simulink model "NonLinear_MotorControl"  (R2017b)
settings: Solver=ode4  StartTime=0.0  StopTime=10  FixedStep=0.0001  MaxStep=0.001  MinStep=0.0001  RelTol=1e-3
(part 2 of 2)

== matlab function NonLinear_MotorControl/System Dynamics/MATLAB Function ==
  data: q input; tau input; q_ddot output; q_dot input
function q_ddot = fcn(q,tau,q_dot)
   q_1 = q(1);
   q_2 = q(2);
   q_3 = q(3);
   q_4 = q(4);
   q_5 = q(5);
   %% M
   M = ...
[                                                                                                                                                                                                                                                                                                                                                                                                                                                                                                                                                                                                                                                                                                                                                                                                               243/2,                                                                                                                                                                                                                               (1637253847765431*cos(q_2 + q_4 + q_5))/2748779069440 + (3015813*sin(q_2 + q_4 + q_5))/12500 + (1637253847765431*cos(q_2 + q_4 - q_5))/2748779069440 + (3015813*sin(q_2 + q_4 - q_5))/12500 - (1637253847765431*cos(q_2 + q_4))/1374389534720 + (13930449*cos(q_2))/500000 + (11396226878722115871*sin(q_2))/1759218604441600 - (1637253847765431*2^(1/2)*cos(q_2 + q_4 - q_5))/2748779069440 - (3015813*2^(1/2)*sin(q_2 + q_4 - q_5))/25000 - (3567380807909369503983*2^(1/2)*cos(q_2 + q_4))/2199023255552000000 + (1637253847765431*2^(1/2)*cos(q_2 + q_4 + q_5))/2748779069440 + (3015813*2^(1/2)*sin(q_2 + q_4 + q_5))/25000,                                                                            0,                                                                                                                                                                                                                                                                                                               (1637253847765431*cos(q_2 + q_4 + q_5))/2748779069440 + (3015813*sin(q_2 + q_4 + q_5))/12500 + (1637253847765431*cos(q_2 + q_4 - q_5))/2748779069440 + (3015813*sin(q_2 + q_4 - q_5))/12500 - (1637253847765431*cos(q_2 + q_4))/1374389534720 - (1637253847765431*2^(1/2)*cos(q_2 + q_4 - q_5))/2748779069440 - (3015813*2^(1/2)*sin(q_2 + q_4 - q_5))/25000 - (3567380807909369503983*2^(1/2)*cos(q_2 + q_4))/2199023255552000000 + (1637253847765431*2^(1/2)*cos(q_2 + q_4 + q_5))/2748779069440 + (3015813*2^(1/2)*sin(q_2 + q_4 + q_5))/25000,                                                                                           (1637253847765431*cos(q_2 + q_4 + q_5))/2748779069440 + (3015813*sin(q_2 + q_4 + q_5))/12500 - (1637253847765431*cos(q_2 + q_4 - q_5))/2748779069440 - (3015813*sin(q_2 + q_4 - q_5))/12500 + (1637253847765431*2^(1/2)*cos(q_2 + q_4 - q_5))/2748779069440 + (3015813*2^(1/2)*sin(q_2 + q_4 - q_5))/25000 + (1637253847765431*2^(1/2)*cos(q_2 + q_4 + q_5))/2748779069440 + (3015813*2^(1/2)*sin(q_2 + q_4 + q_5))/25000
  (13930449*cos(q_2))/500000 + (11396226878722115871*sin(q_2))/1759218604441600 - (1637253847765431*cos(q_2)*cos(q_4))/1374389534720 + (1637253847765431*sin(q_2)*sin(q_4))/1374389534720 - (3567380807909369503983*2^(1/2)*cos(q_2)*cos(q_4))/2199023255552000000 + (3567380807909369503983*2^(1/2)*sin(q_2)*sin(q_4))/2199023255552000000 + (1637253847765431*cos(q_2)*cos(q_4)*cos(q_5))/1374389534720 + (3015813*cos(q_2)*cos(q_5)*sin(q_4))/6250 + (3015813*cos(q_4)*cos(q_5)*sin(q_2))/6250 - (1637253847765431*cos(q_5)*sin(q_2)*sin(q_4))/1374389534720 + (3015813*2^(1/2)*cos(q_2)*cos(q_4)*sin(q_5))/12500 - (1637253847765431*2^(1/2)*cos(q_2)*sin(q_4)*sin(q_5))/1374389534720 - (1637253847765431*2^(1/2)*cos(q_4)*sin(q_2)*sin(q_5))/1374389534720 - (3015813*2^(1/2)*sin(q_2)*sin(q_4)*sin(q_5))/12500,  sin(q_5)/1000 - (47028073017942265058105238873*cos(q_5))/151115727451828646838272 - (1637253847765431*sin(q_4))/1374389534720 - (57*sin(2*q_5))/2000 - (86625503688717695659*2^(1/2)*sin(2*q_5))/2748779069440000 - (3015813*cos(q_4)*cos(q_5))/6250 + (1637253847765431*cos(q_5)*sin(q_4))/1374389534720 - (25261205975153249495668933896699961*cos(q_5)^2)/118059162071741130342400000000 + (21357421969732009*2^(1/2))/549755813888 + (3796988859053507*2^(1/2)*cos(q_5))/549755813888 - (3567380807909369503983*2^(1/2)*sin(q_4))/2199023255552000000 - (86625502314328160939*2^(1/2)*sin(q_5))/1374389534720000 - (16938612281049*2^(1/2)*cos(q_5)^2)/68719476736 + (1637253847765431*2^(1/2)*cos(q_4)*sin(q_5))/1374389534720 + (3015813*2^(1/2)*sin(q_4)*sin(q_5))/12500 + 31233135728824415250615508218939171019991/4835703278458516698824704000000000,                                                                            0, sin(q_5)/1000 - (47028073017942265058105238873*cos(q_5))/151115727451828646838272 - (1637253847765431*sin(q_4))/2748779069440 - (57*sin(2*q_5))/2000 - (86625503688717695659*2^(1/2)*sin(2*q_5))/2748779069440000 - (3015813*cos(q_4)*cos(q_5))/12500 + (1637253847765431*cos(q_5)*sin(q_4))/2748779069440 - (25261205975153249495668933896699961*cos(q_5)^2)/118059162071741130342400000000 + (21357421969732009*2^(1/2))/549755813888 + (3796988859053507*2^(1/2)*cos(q_5))/549755813888 - (3567380807909369503983*2^(1/2)*sin(q_4))/4398046511104000000 - (86625502314328160939*2^(1/2)*sin(q_5))/1374389534720000 - (16938612281049*2^(1/2)*cos(q_5)^2)/68719476736 + (1637253847765431*2^(1/2)*cos(q_4)*sin(q_5))/2748779069440 + (3015813*2^(1/2)*sin(q_4)*sin(q_5))/25000 + 10245887604910058238243681116147296112739/4835703278458516698824704000000000, (1637253847765431*cos(q_4)*sin(q_5))/2748779069440 - (86625463831421188779*sin(q_5))/1374389534720000 - (8712462106215055*cos(q_5))/274877906944 + (3015813*sin(q_4)*sin(q_5))/12500 + (19877377088082943877744654372831289*2^(1/2))/118059162071741130342400000000 - (47028073017942265058105238873*2^(1/2)*cos(q_5))/302231454903657293676544 + (2^(1/2)*sin(q_5))/1000 - (3015813*2^(1/2)*cos(q_4)*cos(q_5))/25000 + (1637253847765431*2^(1/2)*cos(q_5)*sin(q_4))/2748779069440 + 21357421969732009/274877906944
                                                                                                                                                                                                                                                                                                                                                                                                                                                                                                                                                                                                                                                                                                                                                                                                                    0,                                                                                                                                                                                                                                                                                                                                                                                                                                                                                                                                                                                                                                                                                                                                                                                                                                                               0,                                                                      1539/40,                                                                                                                                                                                                                                                                                                                                                                                                                                                                                                                                                                                                                                                                                                                                                                                                                                                               0,                                                                                                                                                                                                                                                                                                                                                                                                                                        (1637253847765431*sin(q_5))/1374389534720 - (3015813*2^(1/2)*cos(q_5))/12500
                                                                                  (1637253847765431*sin(q_2)*sin(q_4))/1374389534720 - (1637253847765431*cos(q_2)*cos(q_4))/1374389534720 - (3567380807909369503983*2^(1/2)*cos(q_2)*cos(q_4))/2199023255552000000 + (3567380807909369503983*2^(1/2)*sin(q_2)*sin(q_4))/2199023255552000000 + (1637253847765431*cos(q_2)*cos(q_4)*cos(q_5))/1374389534720 + (3015813*cos(q_2)*cos(q_5)*sin(q_4))/6250 + (3015813*cos(q_4)*cos(q_5)*sin(q_2))/6250 - (1637253847765431*cos(q_5)*sin(q_2)*sin(q_4))/1374389534720 + (3015813*2^(1/2)*cos(q_2)*cos(q_4)*sin(q_5))/12500 - (1637253847765431*2^(1/2)*cos(q_2)*sin(q_4)*sin(q_5))/1374389534720 - (1637253847765431*2^(1/2)*cos(q_4)*sin(q_2)*sin(q_5))/1374389534720 - (3015813*2^(1/2)*sin(q_2)*sin(q_4)*sin(q_5))/12500, sin(q_5)/1000 - (47028073017942265058105238873*cos(q_5))/151115727451828646838272 - (1637253847765431*sin(q_4))/2748779069440 - (57*sin(2*q_5))/2000 - (86625503688717695659*2^(1/2)*sin(2*q_5))/2748779069440000 - (3015813*cos(q_4)*cos(q_5))/12500 + (1637253847765431*cos(q_5)*sin(q_4))/2748779069440 - (25261205975153249495668933896699961*cos(q_5)^2)/118059162071741130342400000000 + (21357421969732009*2^(1/2))/549755813888 + (3796988859053507*2^(1/2)*cos(q_5))/549755813888 - (3567380807909369503983*2^(1/2)*sin(q_4))/4398046511104000000 - (86625502314328160939*2^(1/2)*sin(q_5))/1374389534720000 - (16938612281049*2^(1/2)*cos(q_5)^2)/68719476736 + (1637253847765431*2^(1/2)*cos(q_4)*sin(q_5))/2748779069440 + (3015813*2^(1/2)*sin(q_4)*sin(q_5))/25000 + 10245887604910058238243681116147296112739/4835703278458516698824704000000000,                                                                            0,                                                                                                                                                                                                                                                                                                               sin(q_5)/1000 - (47028073017942265058105238873*cos(q_5))/151115727451828646838272 - (57*sin(2*q_5))/2000 - (86625503688717695659*2^(1/2)*sin(2*q_5))/2748779069440000 - (25261205975153249495668933896699961*cos(q_5)^2)/118059162071741130342400000000 + (21357421969732009*2^(1/2))/549755813888 + (3796988859053507*2^(1/2)*cos(q_5))/549755813888 - (86625502314328160939*2^(1/2)*sin(q_5))/1374389534720000 - (16938612281049*2^(1/2)*cos(q_5)^2)/68719476736 + 10245887604910058238243681116147296112739/4835703278458516698824704000000000,                                                                                                                                                                                                   (19877377088082943877744654372831289*2^(1/2))/118059162071741130342400000000 - (86625463831421188779*sin(q_5))/1374389534720000 - (8712462106215055*cos(q_5))/274877906944 - (47028073017942265058105238873*2^(1/2)*cos(q_5))/302231454903657293676544 + (2^(1/2)*sin(q_5))/1000 + 21357421969732009/274877906944
                                                                                                                                                                                                                                                                                                                                              (3015813*cos(q_2)*cos(q_4)*sin(q_5))/6250 - (3015813*sin(q_2)*sin(q_4)*sin(q_5))/6250 - (1637253847765431*cos(q_2)*sin(q_4)*sin(q_5))/1374389534720 - (1637253847765431*cos(q_4)*sin(q_2)*sin(q_5))/1374389534720 + (1637253847765431*2^(1/2)*cos(q_2)*cos(q_4)*cos(q_5))/1374389534720 + (3015813*2^(1/2)*cos(q_2)*cos(q_5)*sin(q_4))/12500 + (3015813*2^(1/2)*cos(q_4)*cos(q_5)*sin(q_2))/12500 - (1637253847765431*2^(1/2)*cos(q_5)*sin(q_2)*sin(q_4))/1374389534720,                                                                                                                                                                                                                                                                                                                                                                       (6254725482634281*cos(q_5))/137438953472 - (86625540797235133099*sin(q_5))/1374389534720000 + (1637253847765431*cos(q_4)*sin(q_5))/2748779069440 + (3015813*sin(q_4)*sin(q_5))/12500 + (19877377088082943877744654372831289*2^(1/2))/118059162071741130342400000000 - (47028073017942265058105238873*2^(1/2)*cos(q_5))/302231454903657293676544 - (3015813*2^(1/2)*cos(q_4)*cos(q_5))/25000 + (1637253847765431*2^(1/2)*cos(q_5)*sin(q_4))/2748779069440 + 21357421969732009/274877906944, (1637253847765431*sin(q_5))/1374389534720 - (3015813*2^(1/2)*cos(q_5))/12500,                                                                                                                                                                                                                                                                                                                                                                                                                                                                                                                                                                         (6254725482634281*cos(q_5))/137438953472 - (86625540797235133099*sin(q_5))/1374389534720000 + (19877377088082943877744654372831289*2^(1/2))/118059162071741130342400000000 - (47028073017942265058105238873*2^(1/2)*cos(q_5))/302231454903657293676544 + 21357421969732009/274877906944,                                                                                                                                                                                                                                                                                                                                                                                                        (21357421969732009*2^(1/2))/274877906944 + 19877377088082943877744654372831289/59029581035870565171200000000];
 
   %% C
   C = ...
[ 0,                                            (3015813*cos(q_2 + q_4 + q_5))/12500 - (1637253847765431*sin(q_2 + q_4 + q_5))/2748779069440 + (3015813*cos(q_2 + q_4 - q_5))/12500 - (1637253847765431*sin(q_2 + q_4 - q_5))/2748779069440 + (1637253847765431*sin(q_2 + q_4))/1374389534720 + (11396226878722115871*cos(q_2))/1759218604441600 - (13930449*sin(q_2))/500000 - (3015813*2^(1/2)*cos(q_2 + q_4 - q_5))/25000 + (1637253847765431*2^(1/2)*sin(q_2 + q_4 - q_5))/2748779069440 + (3567380807909369503983*2^(1/2)*sin(q_2 + q_4))/2199023255552000000 + (3015813*2^(1/2)*cos(q_2 + q_4 + q_5))/25000 - (1637253847765431*2^(1/2)*sin(q_2 + q_4 + q_5))/2748779069440, 0, (3015813*cos(q_2 + q_4 + q_5))/12500 - (1637253847765431*sin(q_2 + q_4 + q_5))/2748779069440 + (3015813*cos(q_2 + q_4 - q_5))/12500 - (1637253847765431*sin(q_2 + q_4 - q_5))/2748779069440 + (1637253847765431*sin(q_2 + q_4))/1374389534720 - (3015813*2^(1/2)*cos(q_2 + q_4 - q_5))/25000 + (1637253847765431*2^(1/2)*sin(q_2 + q_4 - q_5))/2748779069440 + (3567380807909369503983*2^(1/2)*sin(q_2 + q_4))/2199023255552000000 + (3015813*2^(1/2)*cos(q_2 + q_4 + q_5))/25000 - (1637253847765431*2^(1/2)*sin(q_2 + q_4 + q_5))/2748779069440, (3015813*cos(q_2 + q_4 + q_5))/12500 - (1637253847765431*sin(q_2 + q_4 + q_5))/2748779069440 + (3015813*cos(q_2 + q_4 - q_5))/12500 - (1637253847765431*sin(q_2 + q_4 - q_5))/2748779069440 - (3015813*2^(1/2)*cos(q_2 + q_4 - q_5))/25000 + (1637253847765431*2^(1/2)*sin(q_2 + q_4 - q_5))/2748779069440 + (3015813*2^(1/2)*cos(q_2 + q_4 + q_5))/25000 - (1637253847765431*2^(1/2)*sin(q_2 + q_4 + q_5))/2748779069440
  0,                                                                                                                                                                                                                                                                                                                                                                                                                                                                                                                                                                                                                                                                            0, 0,                                                                                                                                                                                                                                       (1637253847765431*cos(q_4)*cos(q_5))/2748779069440 - (1637253847765431*cos(q_4))/2748779069440 + (3015813*cos(q_5)*sin(q_4))/12500 - (3567380807909369503983*2^(1/2)*cos(q_4))/4398046511104000000 + (3015813*2^(1/2)*cos(q_4)*sin(q_5))/25000 - (1637253847765431*2^(1/2)*sin(q_4)*sin(q_5))/2748779069440,                       (8712462106215055*sin(q_5))/274877906944 - (86625463831421188779*cos(q_5))/1374389534720000 + (1637253847765431*cos(q_4)*cos(q_5))/2748779069440 + (3015813*cos(q_5)*sin(q_4))/12500 + (2^(1/2)*cos(q_5))/1000 + (47028073017942265058105238873*2^(1/2)*sin(q_5))/302231454903657293676544 + (3015813*2^(1/2)*cos(q_4)*sin(q_5))/25000 - (1637253847765431*2^(1/2)*sin(q_4)*sin(q_5))/2748779069440
  0,                                                                                                                                                                                                                                                                                                                                                                                                                                                                                                                                                                                                                                                                            0, 0,                                                                                                                                                                                                                                                                                                                                                                                                                                                                                                                                                 0,                                                                                                                                                                                                                                                                                                                                              (1637253847765431*cos(q_5))/1374389534720 + (3015813*2^(1/2)*sin(q_5))/12500
  0,                                                                                                                                                                                                                                                                                                                                                                  (1637253847765431*cos(q_4))/2748779069440 - (1637253847765431*cos(q_4)*cos(q_5))/2748779069440 - (3015813*cos(q_5)*sin(q_4))/12500 + (3567380807909369503983*2^(1/2)*cos(q_4))/4398046511104000000 - (3015813*2^(1/2)*cos(q_4)*sin(q_5))/25000 + (1637253847765431*2^(1/2)*sin(q_4)*sin(q_5))/2748779069440, 0,                                                                                                                                                                                                                                                                                                                                                                                                                                                                                                                                                 0,                                                                                                                                                                                                                         (8712462106215055*sin(q_5))/274877906944 - (86625463831421188779*cos(q_5))/1374389534720000 + (2^(1/2)*cos(q_5))/1000 + (47028073017942265058105238873*2^(1/2)*sin(q_5))/302231454903657293676544
  0, (1637253847765431*sin(q_4)*sin(q_5))/2748779069440 - cos(q_5)/1000 - (47028073017942265058105238873*sin(q_5))/302231454903657293676544 - (16938612281049*2^(1/2)*sin(2*q_5))/137438953472 - (3015813*cos(q_4)*sin(q_5))/12500 - (25261205975153249495668933896699961*sin(2*q_5))/236118324143482260684800000000 + (57*cos(q_5)^2)/1000 - (86625543546014202539*2^(1/2))/2748779069440000 + (86625463831421188779*2^(1/2)*cos(q_5))/2748779069440000 - (8712462106215055*2^(1/2)*sin(q_5))/549755813888 + (86625503688717695659*2^(1/2)*cos(q_5)^2)/1374389534720000 - (1637253847765431*2^(1/2)*cos(q_4)*cos(q_5))/2748779069440 - (3015813*2^(1/2)*cos(q_5)*sin(q_4))/25000, 0,                                                                        (57*cos(q_5)^2)/1000 - cos(q_5)/1000 - (47028073017942265058105238873*sin(q_5))/302231454903657293676544 - (16938612281049*2^(1/2)*sin(2*q_5))/137438953472 - (25261205975153249495668933896699961*sin(2*q_5))/236118324143482260684800000000 - (86625543546014202539*2^(1/2))/2748779069440000 + (86625463831421188779*2^(1/2)*cos(q_5))/2748779069440000 - (8712462106215055*2^(1/2)*sin(q_5))/549755813888 + (86625503688717695659*2^(1/2)*cos(q_5)^2)/1374389534720000,                                                                                                                                                                                                                                                                                                                                                                                                                         0];
 
   %% G
   G = ...
[ 
                                                                                      0
                                                                                      0
                                                                          -1509759/4000
                                                                                      0
 (2958512553*2^(1/2)*cos(q_5))/1250000 - (1606146024657887811*sin(q_5))/137438953472000];
   %% Dynamic Calc
   q_ddot = M\(-C*q_dot - G + tau);
end

== matlab function NonLinear_MotorControl/MATLAB Function ==
  settings: updateMethod=DISCRETE
  data: time input; q output; q_dot output; q_ddot output
function [q,q_dot,q_ddot] = TrajectoryPlanner(time)
    x = 350*sin(10*pi/3*time);
    y = -1500*tanh(time/7) - 400;
    z = (x.^2/50 - (y+1000).^2/100)/4 - 1500;
    
    q = inverse_kine(x,y,z);
    persistent q_old q_oold
    if isempty(q_old)
        q_old  = [0;0;0;0;0];
        q_oold = [0;0;0;0;0];
    end
    q_dot = (q - q_old)*10000;
    q_ddot = (q - 2*q_old + q_oold)*100000000;
    
    q_oold = q_old;
    q_old  = q;
end

function q = inverse_kine(X,Y,Z)
    q2 = -asin(X/450);
    q1 = -Y - 450*cos(q2);
    q3 = - 465 - 50 - 2*285 - Z;
    q4 = -q2;
    q5 = 0;
    q = [q1;q2;q3;q4;q5];
end

== matlab function NonLinear_MotorControl/MATLAB Function1 ==
  data: x output; q input; y output; z output
function [x,y,z] = fkine(q)
phi_1 = q(1);
phi_2 = q(2);
phi_3 = q(3);
phi_4 = q(4);
phi_5 = q(5);

T_total = ...
[0.7071*sin(phi_2)*sin(phi_4)*sin(phi_5) - 0.7071*cos(phi_2)*cos(phi_4)*sin(phi_5) - cos(phi_2)*cos(phi_5)*sin(phi_4) - cos(phi_4)*cos(phi_5)*sin(phi_2), 0.1036*cos(phi_2 + phi_4 - phi_5) - 0.6036*cos(phi_2 + phi_4 + phi_5) - 0.5000*cos(phi_2 + phi_4), 0.1036*cos(phi_2 + phi_4 - phi_5) - 0.6036*cos(phi_2 + phi_4 + phi_5) + 0.5000*cos(phi_2 + phi_4),          -450*sin(phi_2)
 0.7071*cos(phi_2)*sin(phi_4)*sin(phi_5) - cos(phi_2)*cos(phi_4)*cos(phi_5) + 0.7071*cos(phi_4)*sin(phi_2)*sin(phi_5) + cos(phi_5)*sin(phi_2)*sin(phi_4), 0.6036*sin(phi_2 + phi_4 + phi_5) - 0.1036*sin(phi_2 + phi_4 - phi_5) + 0.5000*sin(phi_2 + phi_4), 0.6036*sin(phi_2 + phi_4 + phi_5) - 0.1036*sin(phi_2 + phi_4 - phi_5) - 0.5000*sin(phi_2 + phi_4), - phi_1 - 450*cos(phi_2)
                                                                                                                                      -0.7071*sin(phi_5),                                                                        0.5000 - 0.5000*cos(phi_5),                                                                      - 0.5000*cos(phi_5) - 0.5000,           - phi_3 - 1085
                                                                                                                                                       0,                                                                                                 0,                                                                                                 0,                        1];

    
    P = T_total * [0;0;0;1];
    x = P(1);
    y = P(2);
    z = P(3); 
end

== matlab function NonLinear_MotorControl/MATLAB Function2 ==
  data: q_desired input; q_system input; q1 output; q2 output; q3 output; q4 output; q5 output
function [q1,q2,q3,q4,q5] = Plotter(q_desired,q_system)
    q1 = [q_system(1) q_desired(1)];
    q2 = [q_system(2) q_desired(2)];
    q3 = [q_system(3) q_desired(3)];
    q4 = [q_system(4) q_desired(4)];
    q5 = [q_system(5) q_desired(5)];
end

== matlab function NonLinear_MotorControl/MATLAB Function3 ==
  data: x output; q input; y output; z output
function [x,y,z] = fkine(q)
phi_1 = q(1);
phi_2 = q(2);
phi_3 = q(3);
phi_4 = q(4);
phi_5 = q(5);

T_total = ...
[0.7071*sin(phi_2)*sin(phi_4)*sin(phi_5) - 0.7071*cos(phi_2)*cos(phi_4)*sin(phi_5) - cos(phi_2)*cos(phi_5)*sin(phi_4) - cos(phi_4)*cos(phi_5)*sin(phi_2), 0.1036*cos(phi_2 + phi_4 - phi_5) - 0.6036*cos(phi_2 + phi_4 + phi_5) - 0.5000*cos(phi_2 + phi_4), 0.1036*cos(phi_2 + phi_4 - phi_5) - 0.6036*cos(phi_2 + phi_4 + phi_5) + 0.5000*cos(phi_2 + phi_4),          -450*sin(phi_2)
 0.7071*cos(phi_2)*sin(phi_4)*sin(phi_5) - cos(phi_2)*cos(phi_4)*cos(phi_5) + 0.7071*cos(phi_4)*sin(phi_2)*sin(phi_5) + cos(phi_5)*sin(phi_2)*sin(phi_4), 0.6036*sin(phi_2 + phi_4 + phi_5) - 0.1036*sin(phi_2 + phi_4 - phi_5) + 0.5000*sin(phi_2 + phi_4), 0.6036*sin(phi_2 + phi_4 + phi_5) - 0.1036*sin(phi_2 + phi_4 - phi_5) - 0.5000*sin(phi_2 + phi_4), - phi_1 - 450*cos(phi_2)
                                                                                                                                      -0.7071*sin(phi_5),                                                                        0.5000 - 0.5000*cos(phi_5),                                                                      - 0.5000*cos(phi_5) - 0.5000,           - phi_3 - 1085
                                                                                                                                                       0,                                                                                                 0,                                                                                                 0,                        1];

    
    P = T_total * [0;0;0;1];
    x = P(1);
    y = P(2);
    z = P(3); 
end
